simulink model "ame532Project1_onedrive"  (R2023a)
settings: Solver=ode4  StartTime=0.0  StopTime=60  FixedStep=0.01  RelTol=1e-3
model workspace (MAT data in the model file):
  theta : Simulink.Parameter (value not decoded)
undefined symbols (not defined in the file or in its folder): earthRadius
libraries: simulink_extras x11, matrix_library x7, simulink x5, slpidlib x3, aerolibfltsims x2, vrlib x1, aerolibtransform2 x1, aerolibutil x1
(part 2 of 2)

== matlab function ame532Project1_onedrive/9 DoF Dynamic Aircraft model/Unused tranlational kinmatics/C_EN4 ==
  data: roll input; ZYXDCM output; pitch input; yaw input
function ZYXDCM = DCM_from_Euler(roll,pitch,yaw) % sequence is yaw pitch roll
    yaw_matrix = [cos(yaw) sin(yaw) 0;
                  -sin(yaw) cos(yaw) 0;
                  0 0 1];
    pitch_matrix = [cos(pitch) 0 -sin(pitch);
                    0           1           0;
                    sin(pitch) 0  cos(pitch)];
    roll_matrix = [1            0           0;
                    0          cos(roll)    sin(roll);
                    0           -sin(roll)  cos(roll)];
    ZYXDCM = roll_matrix*pitch_matrix*yaw_matrix;
end

== matlab function ame532Project1_onedrive/9 DoF Dynamic Aircraft model/translational dynamics/MATLAB Function10 ==
  data: p input; Cross_Product_Matrix output; q input; r input
function Cross_Product_Matrix = omega_to_cross_product_matrix(p,q,r)

    Cross_Product_Matrix =[0 -r q; r 0 -p; -q p 0];

end

== matlab function ame532Project1_onedrive/9 DoF Dynamic Aircraft model/aeroforce coefficient block/MATLAB Function ==
  data: AR_matrix input; CL_a output
function CL_a = Calculate_CL_a(AR_matrix)

CL_a = zeros(4,1);

for i = 1:4
    CL_a(i) = 2*pi*(AR_matrix(i)/(2+AR_matrix(i)));
end

== matlab function ame532Project1_onedrive/9 DoF Dynamic Aircraft model/aeroforce coefficient block/extract matrix function2 ==
  data: aero_surface_matrix input; Area_matrix output
function Area_matrix = Extract_Area(aero_surface_matrix)

Area_matrix = aero_surface_matrix(:,6);
end

== matlab function ame532Project1_onedrive/9 DoF Dynamic Aircraft model/Translational Kinematics/new C_EN base on cart. coordinate1 ==
  data: lat input; ZYXDCM output; long input
function ZYXDCM = DCM_from_Euler(lat,long) % sequence of rotation is lat long
%     yaw_matrix = [cos(yaw) sin(yaw) 0;
%                   -sin(yaw) cos(yaw) 0;
%                   0 0 1];
    lat_matrix = [cos(lat) 0 -sin(lat);
                    0           1           0;
                    sin(lat) 0  cos(lat)];
    long_matrix = [1            0           0;
                    0          cos(-long)    sin(-long);
                    0           -sin(-long)  cos(-long)];

    adjust_matrix = [cos(pi/2) 0 -sin(pi/2);
                    0           1           0;
                    sin(pi/2) 0  cos(pi/2)];
    ZYXDCM = adjust_matrix*long_matrix*lat_matrix;
end

%this rotational matrix turns lat long coordinate into a new C_EN
%assuming the N CS is lat and longitudinally rotated, then you would do
%-longditudinal rotation then lat rotation, then rotate 90 degrees again to
%match ECEF

== matlab function ame532Project1_onedrive/9 DoF Dynamic Aircraft model/measurement subsystem/MATLAB Function ==
  data: velocity input; magnitude output
function magnitude = magnitude_from_vector(velocity)

magnitude = sqrt(velocity(1)^2+velocity(2)^2+velocity(3)^2);

end

== matlab function ame532Project1_onedrive/9 DoF Dynamic Aircraft model/mass & aero property calculation/CG calculation ==
  data: M_matrix input; cg_x output; cg_y output; cg_z output
function [cg_x, cg_y, cg_z] = CG_calc(M_matrix)

mass_col = M_matrix(:,1);
x_col = M_matrix(:,5);
y_col = M_matrix(:,6);
z_col = M_matrix(:,7);

cg_x = sum(mass_col.*x_col)/(sum(mass_col));
cg_y = sum(mass_col.*y_col)/(sum(mass_col));
cg_z = sum(mass_col.*z_col)/(sum(mass_col));

end

== matlab function ame532Project1_onedrive/9 DoF Dynamic Aircraft model/mass & aero property calculation/MATLAB Function ==
  data: cg_location input; M_matrix input; J_matrix output
function J_matrix = fcn(cg_location,M_matrix)


mass_col = M_matrix(:,1);
x_dim = M_matrix(:,2);
y_dim = M_matrix(:,3);
z_dim = M_matrix(:,4);
x_loc = M_matrix(:,5);
y_loc = M_matrix(:,6);
z_loc = M_matrix(:,7);

Ixx = zeros(11,1);
Iyy = zeros(11,1);
Izz = zeros(11,1);
Ixz = zeros(11,1);
Izx = Ixz;
Ixy = zeros(11,1);
Iyx = Ixy;
Iyz = zeros(11,1);
Izy = Iyz;

J_matrix = zeros(3,3);

% all moment of inertial is calculated wrt to CG

for i = 1:11
    Ixx(i) = mass_col(i)*(y_dim(i)^2+z_dim(i)^2)/(12)+mass_col(i)*((y_loc(i)-cg_location(2))^2+(z_loc(i)-cg_location(3))^2); % check discussion post
    Iyy(i) = mass_col(i)*(x_dim(i)^2+z_dim(i)^2)/(12)+mass_col(i)*((x_loc(i)-cg_location(1))^2+(z_loc(i)-cg_location(3))^2);
    Izz(i) = mass_col(i)*(y_dim(i)^2+x_dim(i)^2)/(12)+mass_col(i)*((y_loc(i)-cg_location(2))^2+(x_loc(i)-cg_location(1))^2);
    Ixz(i) = mass_col(i)*((z_loc(i)-cg_location(3))*(x_loc(i)-cg_location(1)));
    Ixy(i) = mass_col(i)*((x_loc(i)-cg_location(1))*(y_loc(i)-cg_location(2)));
    Iyz(i) = mass_col(i)*((y_loc(i)-cg_location(2))*(z_loc(i)-cg_location(3)));


end

J_matrix(1,1) = sum(Ixx);
J_matrix(2,2) = sum(Iyy);
J_matrix(3,3) = sum(Izz);
J_matrix(1,2) = sum(Ixy);
J_matrix(2,1) = sum(Ixy);
J_matrix(1,3) = sum(Ixz);
J_matrix(3,1) = sum(Ixz);
J_matrix(2,3) = sum(Iyz);
J_matrix(3,2) = sum(Iyz);

J_matrix = J_matrix./1000;
end

== matlab function ame532Project1_onedrive/9 DoF Dynamic Aircraft model/mass & aero property calculation/MATLAB Function2 ==
  data: M_matrix input; aero_prop output
function aero_prop = fcn(M_matrix)

aero_prop = zeros(4,7);
for i = 1:4
    aero_prop(i,1:3) = M_matrix(i,5:7);
    aero_prop(i,4) = M_matrix(i,2);
end

%% define span for each surface

    aero_prop(1,5) = M_matrix(1,3); %right wing
    aero_prop(2,5) = M_matrix(2,3); %left wing
    aero_prop(3,5) = M_matrix(3,3); %hor stab.
    aero_prop(4,5) = M_matrix(4,4); %ver stab.
%% define area and aspect ratio for each surface

for i = 1:4
    aero_prop(i,6) = aero_prop(i,4)*aero_prop(i,5);
    aero_prop(i,7) = aero_prop(i,5)/aero_prop(i,4);
end

== matlab function ame532Project1_onedrive/9 DoF Dynamic Aircraft model/aeroforce coefficient block/extract matrix function ==
  data: aero_surface_matrix input; AR_matrix output
function AR_matrix = Extract_AR(aero_surface_matrix)

AR_matrix = aero_surface_matrix(:,7);
end

== matlab function ame532Project1_onedrive/9 DoF Dynamic Aircraft model/aeroforce coefficient block/calculatie alpha ==
  data: i0 input; alpha output; v_B input; n_vector input; wind_w input; v_B_BA output; C_BN input
function [alpha,v_B_BA] = fcn(i0,v_B,n_vector,wind_w,C_BN)

alpha = zeros(4,1);
% this function calculates alpha that the aero surface sees

v_B_BA = v_B - C_BN*wind_w;

for i = 1:4
    alpha(i) = i0(i) - asin(dot(v_B_BA,n_vector(:,i))/norm(v_B_BA));
end

== matlab function ame532Project1_onedrive/9 DoF Dynamic Aircraft model/aeroforce coefficient block/MATLAB Function1 ==
  data: CL0 input; CL_s output; CL_a input; alpha input; surface_area input; deflection_angle input
function CL_s = calculate_CL_s(CL0,CL_a,alpha,surface_area,deflection_angle)

CL_s = zeros(4,1);

for i = 1:4
    CL_s(i) = CL0(i)+CL_a(i)*alpha(i)+3*deflection_angle(i)*(0.3);
end

== matlab function ame532Project1_onedrive/9 DoF Dynamic Aircraft model/Rotational Kinematics/MATLAB Function2 ==
  data: phi input; H_matrix_inv output; theta input; psi input
function H_matrix_inv = inv_h_matrix_from_euler(phi,theta,psi)

H_matrix_inv = [1, tan(theta)*sin(phi), tan(theta)*cos(phi);
                0,      cos(phi),           -sin(phi);      
                0,     sin(phi)/cos(theta),   cos(phi)/cos(theta)];

end

== matlab function ame532Project1_onedrive/9 DoF Dynamic Aircraft model/aeroforce coefficient block/MATLAB Function2 ==
  data: CD_0 input; CD_a input; CD_s output; alpha_0 input; alpha input; CL_s input; e input; AR input
function CD_s = calculate_CD_s(CD_0,CD_a,alpha_0,alpha,CL_s,e,AR)
CD_s = zeros(4,1);

for i = 1:4
    
    CD_s(i) = CD_0(i) + CD_a(i)*(alpha(i)-alpha_0(i))^2+(CL_s(i)^2)/(pi*e(i)*AR(i));

end

== matlab function ame532Project1_onedrive/9 DoF Dynamic Aircraft model/aeroforce coefficient block/extract matrix function1 ==
  data: aero_surface_matrix input; AR_matrix output
function AR_matrix = Extract_AR(aero_surface_matrix)

AR_matrix = aero_surface_matrix(:,7);
end

== matlab function ame532Project1_onedrive/9 DoF Dynamic Aircraft model/aeroforce coefficient block/MATLAB Function3 ==
  data: alpha input; CM_0 input; CM_s output; CM_a input
function CM_s = calculate_CM_s(alpha,CM_0,CM_a)

CM_s = zeros(4,1);

for i = 1:4
    CM_s(i) = CM_0(i)+CM_a(i)*alpha(i);
end

== matlab function ame532Project1_onedrive/9 DoF Dynamic Aircraft model/aeroforce & moment block/MATLAB Function ==
  data: CL_s input; Lift_s output; totalspeed input; area_s input
function Lift_s = calculate_Lift_s(CL_s,totalspeed,area_s)

Lift_s = zeros(4,1);
rho = 1.225; %kg/m3

for i = 1:4
    Lift_s(i) = CL_s(i)*0.5*rho*(totalspeed^2)*area_s(i);
end

end

== matlab function ame532Project1_onedrive/9 DoF Dynamic Aircraft model/aeroforce & moment block/MATLAB Function1 ==
  data: aerosurface_matrix input; area_col output
function area_col = extract_area_col(aerosurface_matrix)

area_col = aerosurface_matrix(:,6);

end

== matlab function ame532Project1_onedrive/9 DoF Dynamic Aircraft model/aeroforce & moment block/MATLAB Function2 ==
  data: CD_s input; Drag_s output; totalspeed input; area_s input
function Drag_s = calculate_Drag_s(CD_s,totalspeed,area_s)

Drag_s = zeros(4,1);
rho = 1.225; %kg/m3

for i = 1:4
    Drag_s(i) = CD_s(i)*0.5*rho*(totalspeed^2)*area_s(i);
end

end

== matlab function ame532Project1_onedrive/9 DoF Dynamic Aircraft model/aeroforce & moment block/MATLAB Function3 ==
  data: CM_s input; Moment_s output; totalspeed input; area_s input; chord_s input
function Moment_s = calculate_Moment_s(CM_s,totalspeed,area_s,chord_s)

Moment_s = zeros(4,1);
rho = 1.225; %kg/m3

for i = 1:4
    Moment_s(i) = CM_s(i)*0.5*rho*(totalspeed^2)*area_s(i)*chord_s(i);
end

end

== matlab function ame532Project1_onedrive/9 DoF Dynamic Aircraft model/aeroforce & moment block/MATLAB Function4 ==
  data: aerosurface_matrix input; chord_col output
function chord_col = extract_chord_col(aerosurface_matrix)

chord_col = aerosurface_matrix(:,4);

end

== matlab function ame532Project1_onedrive/9 DoF Dynamic Aircraft model/aeroforce & moment block/MATLAB Function5 ==
  data: Lift_s input; F_w_s output; n_vector_s input; Drag_s input
function F_w_s = Calculate_F_w(Lift_s,n_vector_s,Drag_s)

F_w_s = zeros(3,4);

for i = 1:4
    F_w_s(:,i) = Lift_s(i).*n_vector_s(:,i) - [Drag_s(i) 0 0]';
end

== matlab function ame532Project1_onedrive/9 DoF Dynamic Aircraft model/aeroforce & moment block/MATLAB Function6 ==
  data: n_vector_s input; M_s input; M_w_s output; F_b_s input; x_b_sb input
function M_w_s = Calculate_M_w(n_vector_s,M_s,F_b_s,x_b_sb)

M_w_s = zeros(3,4);

for i = 1:4
      M_w_s(:,i) = M_s(i)*[0 0 0; 0 0 -1; 0 1 0]*n_vector_s(:,i)+cross(x_b_sb(:,i),F_b_s(:,i));
%     M_w_s(:,i) = M_s(i)*[0 0 0; 0 0 -1; 0 1 0]*n_vector_s(:,i)+cross(F_b_s(:,i),x_b_sb(:,i));

end

== matlab function ame532Project1_onedrive/9 DoF Dynamic Aircraft model/Rotational Kinematics/MATLAB Function3 ==
  data: p input; Cross_Product_Matrix output; q input; r input
function Cross_Product_Matrix = omega_to_cross_product_matrix(p,q,r)

    Cross_Product_Matrix =[0 -r q; r 0 -p; -q p 0];

end

== matlab function ame532Project1_onedrive/9 DoF Dynamic Aircraft model/mass & aero property calculation/MATLAB Function1 ==
  data: aero_prop_matrix input; m_matrix input; x_b_s_ac output; cg_location input
function x_b_s_ac = calculate_x_b_sb(aero_prop_matrix,m_matrix,cg_location)
%this function calculates vector of each component to CM of aircraft

x_b_sb = zeros(3,4);
x_b_s_ac = zeros(3,4);
for i = 1:4
    x_b_s_ac(:,i) = m_matrix(i,5:7)' + [0.25*aero_prop_matrix(i,4) 0 0]';
    x_b_s_ac(:,i) = x_b_s_ac(:,i)- cg_location;

%     x_b_sb(:,i) = m_matrix(i,5:7)' - cg_location;

end

== matlab function ame532Project1_onedrive/9 DoF Dynamic Aircraft model/aeroforce & moment block/MATLAB Function7 ==
  data: forcexyz_w_s_matrix input; force_xyz_w output
function force_xyz_w = sum_all_force_xyz(forcexyz_w_s_matrix)

force_xyz_w = zeros(3,1);

for i = 1:3
    force_xyz_w(i) = sum(forcexyz_w_s_matrix(i,:));
end

== matlab function ame532Project1_onedrive/9 DoF Dynamic Aircraft model/aeroforce & moment block/MATLAB Function8 ==
  data: m_b_s input; moments_lmn_b output
function moments_lmn_b = sum_all_moments_b_s(m_b_s)

moments_lmn_b = zeros(3,1);

for i = 1:3
    moments_lmn_b(i) = sum(m_b_s(i,:));
end

== matlab function ame532Project1_onedrive/9 DoF Dynamic Aircraft model/aeroforce & moment block/MATLAB Function9 ==
  data: DCM_WB output; v_body_ba input; alpha output; beta output; v_inf output
function [DCM_WB,alpha,beta,v_inf]  = construct_DCM_bw(v_body_ba)

alpha = atan2(v_body_ba(3),v_body_ba(1));
beta = asin(v_body_ba(2)/norm(v_body_ba));

DCM_WB = [cos(beta) sin(beta) 0; -sin(beta) cos(beta) 0; 0 0 1]*[cos(alpha) 0 sin(alpha); 0 1 0; -sin(alpha) 0 cos(alpha)];
v_inf = norm(v_body_ba);
end

== matlab function ame532Project1_onedrive/9 DoF Dynamic Aircraft model/Rotational Kinematics/MATLAB Function4 ==
  data: DCM input; roll output; pitch output; yaw output
function [roll, pitch, yaw] = Euler_from_DCM(DCM)
   roll = atan2(DCM(2,3),DCM(3,3));
   pitch = -asin(DCM(1,3));
   yaw = atan2(DCM(1,2),DCM(1,1));
end

== matlab function ame532Project1_onedrive/9 DoF Dynamic Aircraft model/Rotational Kinematics/C_EN1 ==
  data: roll input; ZYXDCM output; pitch input; yaw input
function ZYXDCM = DCM_from_Euler(roll,pitch,yaw) % sequence is yaw pitch roll
    yaw_matrix = [cos(yaw) sin(yaw) 0;
                  -sin(yaw) cos(yaw) 0;
                  0 0 1];
    pitch_matrix = [cos(pitch) 0 -sin(pitch);
                    0           1           0;
                    sin(pitch) 0  cos(pitch)];
    roll_matrix = [1            0           0;
                    0          cos(roll)    sin(roll);
                    0           -sin(roll)  cos(roll)];
    ZYXDCM = roll_matrix*pitch_matrix*yaw_matrix;
end

== matlab function ame532Project1_onedrive/9 DoF Dynamic Aircraft model/Rotational Kinematics/C_EN2 ==
  data: roll input; ZYXDCM output; pitch input; yaw input
function ZYXDCM = DCM_from_Euler(roll,pitch,yaw) % sequence is yaw pitch roll
    yaw_matrix = [cos(yaw) -sin(yaw) 0;
                  sin(yaw) cos(yaw) 0;
                  0 0 1];
    pitch_matrix = [cos(pitch) 0 sin(pitch);
                    0           1           0;
                    -sin(pitch) 0  cos(pitch)];
    roll_matrix = [1            0           0;
                    0          cos(roll)    -sin(roll);
                    0           sin(roll)  cos(roll)];
    ZYXDCM = roll_matrix*pitch_matrix*yaw_matrix;
end

== matlab function ame532Project1_onedrive/9 DoF Dynamic Aircraft model/Rotational Kinematics/MATLAB Function5 ==
  data: DCM input; roll output; pitch output; yaw output
function [roll, pitch, yaw] = Euler_from_DCM(DCM)
   roll = atan2(DCM(2,3),DCM(3,3));
   pitch = asin(DCM(1,3));
   yaw = atan2(DCM(1,2),DCM(1,1));
end

== matlab function ame532Project1_onedrive/9 DoF Dynamic Aircraft model/Rotational Kinematics/MATLAB Function6 ==
  data: DCM input; roll output; pitch output; yaw output
function [roll, pitch, yaw] = Euler_from_DCM(DCM)
   roll = atan2(DCM(2,3),DCM(3,3));
   pitch = -asin(DCM(1,3));
   yaw = atan2(DCM(1,2),DCM(1,1));
end

== matlab function ame532Project1_onedrive/9 DoF Dynamic Aircraft model/Rotational Kinematics/MATLAB Function7 ==
  data: quat input; roll output; pitch output; yaw output
function [roll, pitch, yaw] = Euler_from_Quat(quat)
    DCM = zeros(3,3);
    DCM(1) = (quat(1)^2+quat(2)^2-quat(3)^2-quat(4)^2);
    DCM(2) = 2*(quat(2)*quat(3)-quat(1)*quat(4));
    DCM(3) = 2*(quat(2)*quat(4)+quat(1)*quat(3));
    DCM(4) = 2*(quat(2)*quat(3)+quat(1)*quat(4));
    DCM(5) = (quat(1)^2-quat(2)^2+quat(3)^2-quat(4)^2);
    DCM(6) = 2*(quat(3)*quat(4)-quat(1)*quat(2));
    DCM(7) = 2*(quat(2)*quat(4)-quat(1)*quat(3));
    DCM(8) = 2*(quat(3)*quat(4)+quat(1)*quat(2));
    DCM(9) = (quat(1)^2-quat(2)^2-quat(3)^2+quat(4)^2);

    roll = atan2(DCM(2,3),DCM(3,3));
    pitch = -asin(DCM(1,3));
    yaw = atan2(DCM(1,2),DCM(1,1));
end

== matlab function ame532Project1_onedrive/9 DoF Dynamic Aircraft model/Rotational Kinematics/C_BN ==
  data: roll input; ZYXDCM output; pitch input; yaw input
function ZYXDCM = DCM_from_Euler(roll,pitch,yaw) % sequence is yaw pitch roll
    yaw_matrix = [cos(yaw) sin(yaw) 0;
                  -sin(yaw) cos(yaw) 0;
                  0 0 1];
    pitch_matrix = [cos(pitch) 0 -sin(pitch);
                    0           1           0;
                    sin(pitch) 0  cos(pitch)];
    roll_matrix = [1            0           0;
                    0          cos(roll)    sin(roll);
                    0           -sin(roll)  cos(roll)];
    ZYXDCM = roll_matrix*pitch_matrix*yaw_matrix;
end
